simulink model "rtos"  (R2020b)
settings: Solver=VariableStepAuto  StartTime=0.0  StopTime=Inf  RelTol=1e-3
undefined symbols (not defined in the file): Serial_Port, Standard_Devices
libraries: sldrtlib x1
settings Model: Creator=Utente  LastModifiedBy=Utente

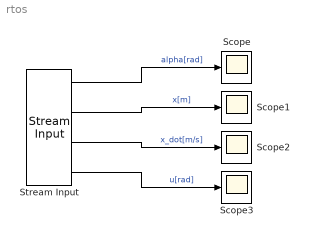
== system rtos ==
  Scope{,1..3} (4 alike) : Scope
  Stream Input : sldrtlib/Stream Input  SampleTime=0.002  MaxMissedTicks=1000  ShowMissedTicks=off  YieldWhenWaiting=off  DrvName=Standard_Devices/Serial_Port  DrvAddress=3  DrvOptions=[115200 8 0 0 0 0 0 0]  DataTypes={'double', 'double', 'double', 'double'}  FormatString='%f,%f,%f,%f'  Terminator={'\r', '\n'}  ShowReady=off  ShowError=off
      settings: AttributesFormatString=Serial Port [3]  SourceProductBaseCode=WT
  wires:
  Stream Input/1 -> Scope/1  "alpha[rad]"
  Stream Input/2 -> Scope1/1  "x[m]"
  Stream Input/3 -> Scope2/1  "x_dot[m/s]"
  Stream Input/4 -> Scope3/1  "u[rad]"
